simulink model "matrixalgorithm"  (R2016b)
settings: Solver=VariableStepAuto  StartTime=0.0  StopTime=200  RelTol=1e-3
values from neighbouring files (symbols this model uses):
  r = 6371    [earth_mag.m]
undefined symbols (not defined in the file or in its folder): I, Kd, Kp, t_limit, w_max
libraries: simulink x1
settings Model: Creator=Evan  LastModifiedBy=Evan

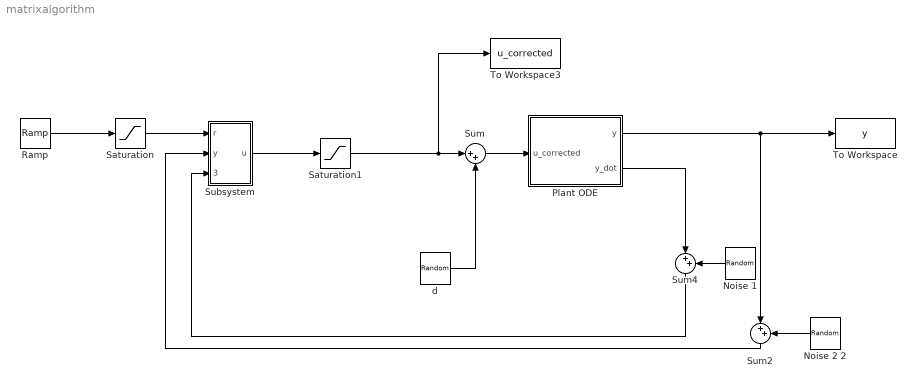
== system matrixalgorithm ==
  Noise 1 : UniformRandomNumber  Minimum=-1e-8  Maximum=.1e-8  SampleTime=0.1
  Noise 2 2 : UniformRandomNumber  Minimum=-1e-8  Maximum=.1e-8  SampleTime=0.1
  "Plant ODE " : Subsystem
  Ramp : simulink/Sources/Ramp  slope=[w_max(1); w_max(2); w_max(3)]  start=0  X0=0
  Saturation : Saturate  UpperLimit=[r(1); r(2); r(3)]  LowerLimit=[-r(1); -r(2); -r(3)]
  Saturation1 : Saturate  UpperLimit=[t_limit(1); t_limit(2); t_limit(3)]  LowerLimit=[-t_limit(1); -t_limit(2); -t_limit(3)]
  Subsystem : Subsystem
  Sum : Sum  Inputs=|++
  Sum2 : Sum  Inputs=|++
  Sum4 : Sum  Inputs=|++
  To Workspace : ToWorkspace  VariableName=y  SaveFormat=Timeseries  SampleTime=-1
  To Workspace3 : ToWorkspace  VariableName=u_corrected  SaveFormat=Timeseries  SampleTime=-1
  "d " : UniformRandomNumber  Minimum=-1e-8  Maximum=.1e-8  SampleTime=0.1
  wires:
  Ramp/1 -> Saturation/1
  Saturation/1 -> Subsystem/1(r)
  Subsystem/1("u ") -> Saturation1/1
  Sum/1 -> "Plant ODE "/1(u_corrected)
  "d "/1 -> Sum/2
  Saturation1/1 -> To Workspace3/1, Sum/1
  Noise 1/1 -> Sum4/2
  "Plant ODE "/2(y_dot) -> Sum4/1
  Sum4/1 -> Subsystem/3("y_dot ")
  Sum2/1 -> Subsystem/2(y)
  "Plant ODE "/1(y) -> To Workspace/1, Sum2/1
  Noise 2 2/1 -> Sum2/2

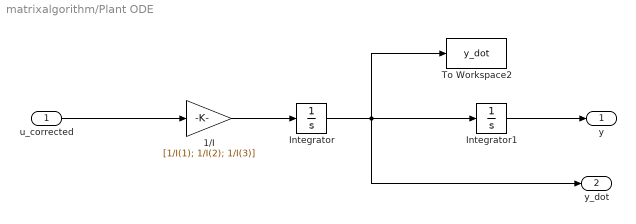
== system matrixalgorithm/Plant ODE  ==
  u_corrected : Inport
  "1/I " : Gain  Gain=[1/I(1); 1/I(2); 1/I(3)]
  Integrator : Integrator
  Integrator1 : Integrator
  To Workspace2 : ToWorkspace  VariableName=y_dot  SaveFormat=Timeseries  SampleTime=-1
  y : Outport
  y_dot : Outport  Port=2
  wires:
  u_corrected/1 -> "1/I "/1
  Integrator/1 -> y_dot/1, Integrator1/1, To Workspace2/1
  Integrator1/1 -> y/1
  "1/I "/1 -> Integrator/1

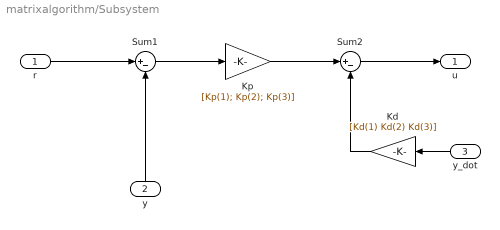
== system matrixalgorithm/Subsystem ==
  r : Inport
  y : Inport  Port=2
  "y_dot " : Inport  Port=3
  "Kd " : Gain  Gain=[Kd(1) Kd(2) Kd(3)]
  "Kp " : Gain  Gain=[Kp(1); Kp(2); Kp(3)]
  Sum1 : Sum  Inputs=|+-
  Sum2 : Sum  Inputs=|+-
  "u " : Outport
  wires:
  Sum1/1 -> "Kp "/1
  Sum2/1 -> "u "/1
  "y_dot "/1 -> "Kd "/1
  y/1 -> Sum1/2
  "Kp "/1 -> Sum2/1
  r/1 -> Sum1/1
  "Kd "/1 -> Sum2/2
